simulink model "Detumbling"  (R2024a)
settings: Solver=VariableStepAuto  StartTime=0.0  StopTime=10.0  RelTol=1e-3
undefined symbols (not defined in the file): k_Bdot
libraries: matrix_library x2
settings Model: Creator=dani  LastModifiedBy=dani

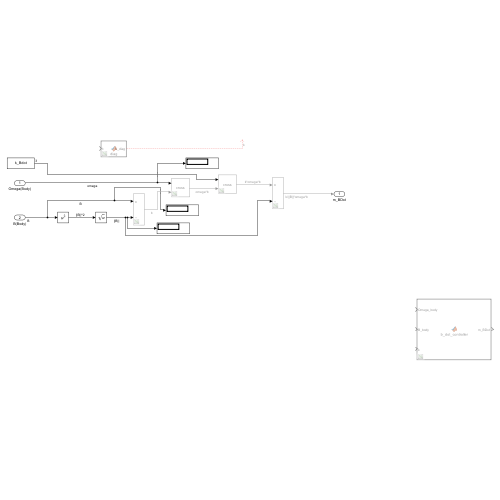
[thumbnail: Simulink's stored preview of the top-level diagram]
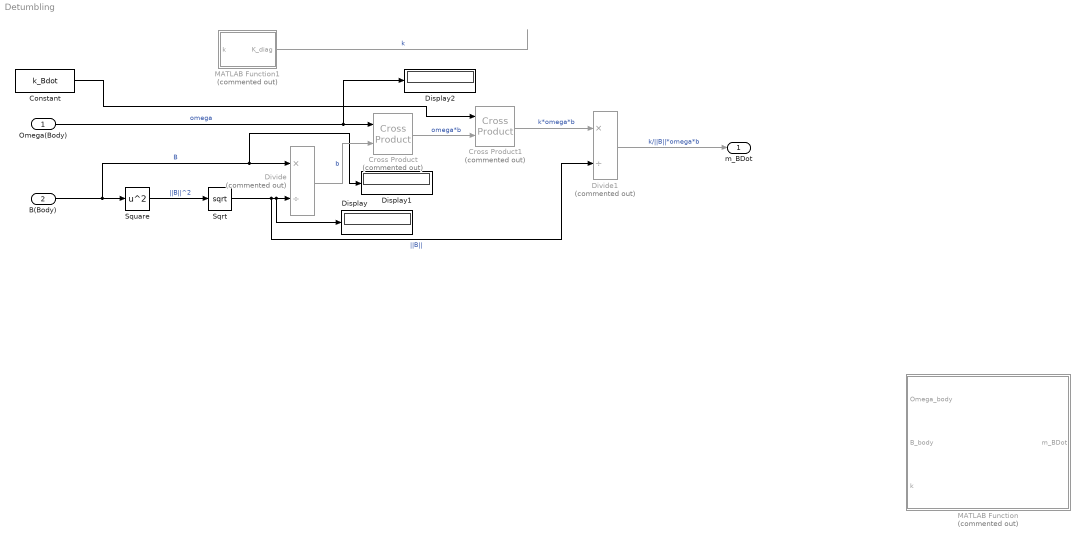
== system Detumbling ==
  Omega(Body) : Inport
  B(Body) : Inport  Port=2
  Constant : Constant  Value=k_Bdot
  Cross Product : matrix_library/Cross Product  Commented=on
  Cross Product1 : matrix_library/Cross Product  Commented=on
  Display : Display
  Display1 : Display
  Display2 : Display
  Divide : Product  Commented=on  Inputs=*/
  Divide1 : Product  Commented=on  Inputs=*/
  MATLAB Function : MATLAB Function  Commented=on  TreatAsAtomicUnit=on
  MATLAB Function1 : MATLAB Function  Commented=on  TreatAsAtomicUnit=on
  Sqrt : Sqrt
  Square : Math  Operator=square
  m_BDot : Outport
  wires:
  Constant/1 -> Cross Product1/1
  Omega(Body)/1 -> Display2/1, Cross Product/1  "omega"
  B(Body)/1 -> Display1/1, Divide/1, Square/1  "B"
  Cross Product/1 -> Cross Product1/2  "omega*b"
  Square/1 -> Sqrt/1  "||B||^2"
  Sqrt/1 -> Divide1/2, Display/1, Divide/2  "||B||"
  Divide/1 -> Cross Product/2  "b"
  MATLAB Function1/1(K_diag) -> ?  "k"
  Cross Product1/1 -> Divide1/1  "k*omega*b"
  Divide1/1 -> m_BDot/1  "k/||B||*omega*b"

== matlab function Detumbling/MATLAB Function1 ==
  data: k input; K_diag output
function K_diag = diag(k)
    K_diag = diag(k);
end

== matlab function Detumbling/MATLAB Function ==
  data: Omega_body input; m_BDot output; B_body input; k input
function m_BDot = b_dot_controller(Omega_body, B_body, k)
    % B-dot controller with axis-specific gains for detumbling
    % m = (1 / ||B||^2) * diag(k) * (w x B)
    
    % Validate that inputs have exactly three elements
    if numel(Omega_body) ~= 3 || numel(B_body) ~= 3 || numel(k) ~= 3
        error('Omega_body, B_body, and k must each have exactly 3 elements.');
    end

    % Calculate the squared magnitude of the magnetic field vector
    B_norm_sq = norm(B_body)^2;

    % Avoid division by zero (set m_BDot to zero if ||B|| is zero)
    if B_norm_sq == 0
        m_BDot = [0; 0; 0];
        return;
    end

    % Compute the cross product: Omega_body x B_body
    cross_w_B = cross(Omega_body, B_body);

    % Apply axis-specific gains and compute the magnetic dipole moment
    m_BDot = (1 / B_norm_sq) * diag(k) * cross_w_B;

    % Ensure output is a column vector
    m_BDot = m_BDot(:);
end
